simulink model "Cruise_ctrl"  (R2020b)
settings: Solver=VariableStepAuto  StartTime=0.0  StopTime=10.0  RelTol=1e-3
values from neighbouring files (symbols this model uses):
  b = 50    [values.m]
  m = 1000    [values.m]
settings Model: DataDictionary=cruisecontrol.sldd  Creator=Abhinav dixit  LastModifiedBy=Abhinav dixit

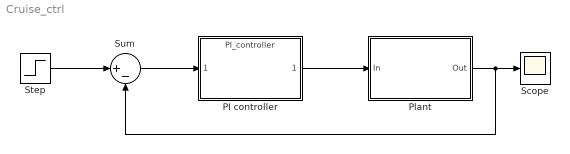
== system Cruise_ctrl ==
  PI controller : ModelReference  ModelNameDialog=PI_controller  SimulationMode=Normal  ModelReferenceVersion=1.2
  Plant : Subsystem
  Scope : Scope
  Step : Step  Time=0  After=u  SampleTime=0
  Sum : Sum  Inputs=|+-
  wires:
  PI controller/1 -> Plant/1(In)
  Plant/1(Out) -> Sum/2, Scope/1
  Sum/1 -> PI controller/1
  Step/1 -> Sum/1

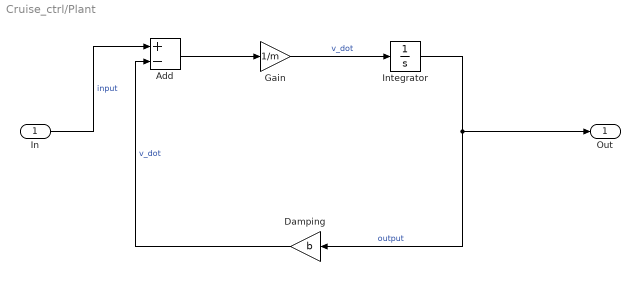
== system Cruise_ctrl/Plant ==
  In : Inport
  Add : Sum  Inputs=+-
  Damping : Gain  Gain=b
  Gain : Gain  Gain=1/m
  Integrator : Integrator
  Out : Outport
  wires:
  Integrator/1 -> Out/1, Damping/1  "output"
  Damping/1 -> Add/2  "v_dot"
  Add/1 -> Gain/1
  In/1 -> Add/1  "input"
  Gain/1 -> Integrator/1  "v_dot"
